simulink model "Redo7LongNoise"  (R2017b)
settings: Solver=ode45  StartTime=0.0  StopTime=MaxTime  MaxStep=timeStep  RelTol=rel  AbsTol=abs  EnableMultiTasking=on
values from neighbouring files (symbols this model uses):
  a0L = asin(min(1,(y0-yG)/l0))    [BigSweep2.m]    (also in NoiseAmbient.m; TheGoodBand.m)
  a0R = a0L-phi0    [BigSweep2.m]    (also in NoiseAmbient.m; TheGoodBand.m)
  g = 9.81    [BigSweep2.m]    (also in ElasticPendulum2.m; NoiseAmbient.m; Original_running_params.m; TheGoodBand.m)
  kL = 12000    [BigSweep2.m]    (also in NoiseAmbient.m; TheGoodBand.m)
  l0 = 1    [BigSweep2.m]    (also in ElasticPendulum2.m; NoiseAmbient.m; Original_running_params.m; TheGoodBand.m)
  m = 80    [BigSweep2.m]    (also in ElasticPendulum2.m; NoiseAmbient.m; Original_running_params.m; TheGoodBand.m)
  NoiseLevel = minNoise+(maxNoise-minNoise)*nNoise/nNoiseRuns+.00000001    [NoiseAmbient.m]    (also in TheGoodBand.m = 1e-08)
  time = now    [NoiseAmbient.m]    (also in TheGoodBand.m)
  Vx0 = real((2/m*(Esys-m*g*(y0-yG)))^.5)    [BigSweep2.m]    (also in ElasticPendulum2.m = 2.11026064741; NoiseAmbient.m = 2.11; TheGoodBand.m = 2.11)
  Vy0 = 0    [BigSweep2.m]    (also in ElasticPendulum2.m; NoiseAmbient.m; TheGoodBand.m)
  x0 = []    [AnimSMR.m]    (also in BigSweep2.m = 3; ElasticPendulum2.m = -0.2; NoiseAmbient.m = 3; Original_running_params.m = 0)
  xL0 = x0+l0*cos(a0L)    [BigSweep2.m]    (also in NoiseAmbient.m; TheGoodBand.m)
  xR0 = x0+l0*cos(a0R)    [BigSweep2.m]    (also in NoiseAmbient.m; TheGoodBand.m)
  y0 = Y0minEver+(yMaxRel-Y0minEver)*NyCycle/Ny    [BigSweep2.m]    (also in ElasticPendulum2.m = 0.98; NoiseAmbient.m = 0.98; Original_running_params.m = 1; TheGoodBand.m = 0.98)
  yG = 0    [BigSweep2.m]    (also in ElasticPendulum2.m; NoiseAmbient.m; Original_running_params.m; TheGoodBand.m)
  yL0 = y0-l0*sin(a0L)    [BigSweep2.m]    (also in NoiseAmbient.m; TheGoodBand.m)
  yR0 = y0-l0*sin(a0R)    [BigSweep2.m]    (also in NoiseAmbient.m; TheGoodBand.m)
libraries: dspswit3 x2, simulink_extras x2
settings Model: Creator=hgeyer  LastModifiedBy=jfr
settings DataIOCC: LimitDataPoints=on  SaveFormat=Array
settings OptimizationCC: ExpressionDepthLimit=2147483647  LifeSpan=inf
settings DebuggingCC: AlgebraicLoopMsg=none  UnderspecifiedInitializationDetection=Classic  MergeDetectMultiDrivingBlocksExec=none  MaxConsecutiveZCsMsg=none  SolverPrmCheckMsg=warning  StateNameClashWarn=warning  SFUnexpectedBacktrackingDiag=warning  SFNoUnconditionalDefaultTransitionDiag=warning  SFExecutionAtInitializationDiag=none
settings HardwareCC: ProdBitPerPointer=32  ProdBitPerSizeT=32  ProdBitPerPtrDiffT=32  ProdLargestAtomicFloat=None  ProdIntDivRoundTo=Undefined  ProdEndianess=Unspecified  ProdWordSize=32  ProdHWDeviceType=32-bit Generic
settings ModelReferenceCC: ModelReferenceMinAlgLoopOccurrences=on  PropagateSignalLabelsOutOfModel=off
settings CodeAppCC: StateflowObjectComments=on
settings GRTTargetCC: TargetLangStandard=C89/C90 (ANSI)  GeneratePreprocessorConditionals=Disable all
settings ConfigComp: CovMetricSettings=dw  CovHtmlReporting=on  CovSaveCumulativeToWorkspaceVar=on  CovSaveSingleToWorkspaceVar=on  CovExternalEMLEnable=off

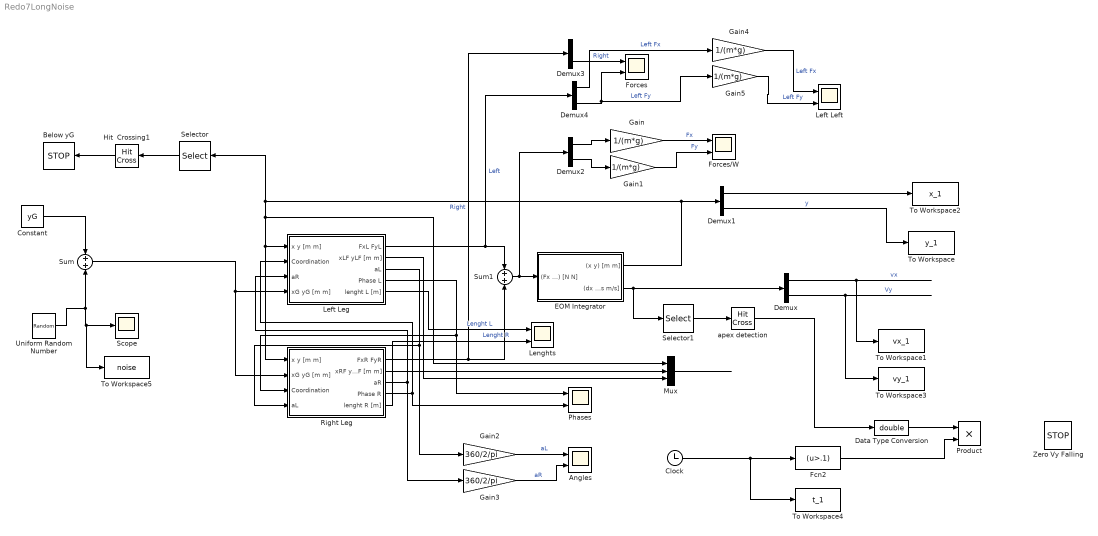
== system Redo7LongNoise ==
  "Angles " : Scope  NumInputPorts=2
  Below yG : Stop
  Clock : Clock
  Constant : Constant  Value=yG
  Data Type Conversion : DataTypeConversion  OutDataTypeStr=double
  Demux{,1..4} (5 alike) : Demux  Outputs=2
  EOM Integrator : Subsystem
  Fcn2 : Fcn  Expr=(u>.1)
  Forces : Scope  NumInputPorts=2
  Forces/W : Scope  NumInputPorts=2
  Gain{,1,4..5} (4 alike) : Gain  Gain=1/(m*g)
  Gain2 : Gain  Gain=360/2/pi
  Gain3 : Gain  Gain=360/2/pi
  Hit  Crossing1 : HitCross  HitCrossingOffset=yG  HitCrossingDirection=falling
  Left Left : Scope  NumInputPorts=2
  Left Leg : Subsystem
  Lenghts : Scope  NumInputPorts=2
  Mux : Mux  Inputs=3
  Phases : Scope  NumInputPorts=2
  Product : Product
  Right Leg : Subsystem
  Scope : Scope
  Selector : Selector  InputPortWidth=2  IndexOptions=Index vector (dialog)  Indices=2  OutputSizes=1
  Selector1 : Selector  InputPortWidth=2  IndexOptions=Index vector (dialog)  Indices=2  OutputSizes=1
  Sum : Sum
  Sum1 : Sum
  To Workspace : ToWorkspace  VariableName=y_1  SampleTime=-1
      settings: MaxDataPoints=1
  To Workspace1 : ToWorkspace  VariableName=vx_1  SampleTime=-1
      settings: MaxDataPoints=1
  To Workspace2 : ToWorkspace  VariableName=x_1  SampleTime=-1
      settings: MaxDataPoints=1
  To Workspace3 : ToWorkspace  VariableName=vy_1  SampleTime=-1
      settings: MaxDataPoints=1
  To Workspace4 : ToWorkspace  VariableName=t_1  SampleTime=-1
      settings: MaxDataPoints=1
  To Workspace5 : ToWorkspace  VariableName=noise  SampleTime=-1
  Uniform Random Number : UniformRandomNumber  Minimum=-NoiseLevel  Maximum=NoiseLevel  Seed=time  SampleTime=0.1
  Zero Vy Falling : Stop
  apex detection : HitCross  HitCrossingDirection=falling
  wires:
  Mux/1 -> ?
  Demux/2 -> To Workspace3/1  "Vy"
  Demux1/2 -> To Workspace/1  "y"
  Demux/1 -> To Workspace1/1  "vx"
  Demux1/1 -> To Workspace2/1
  Constant/1 -> Sum/1
  Left Leg/2(xLF yLF [m m]) -> Mux/3
  Sum/1 -> Left Leg/4(xG yG [m m]), Right Leg/2(xG yG [m m])
  Right Leg/2(xRF yRF [m m]) -> Mux/2
  Sum1/1 -> Demux2/1, EOM Integrator/1((Fx Fy) [N N])
  Gain/1 -> Forces/W/1  "Fx"
  Gain1/1 -> Forces/W/2  "Fy"
  Demux2/1 -> Gain/1
  Demux2/2 -> Gain1/1
  Left Leg/1(FxL FyL) -> Sum1/1, Demux4/1  "Left"
  Demux3/2 -> Forces/1  "Right"
  Gain5/1 -> Left Left/2  "Left Fy"
  Right Leg/1(FxR FyR) -> Sum1/2, Demux3/1  "Right"
  Hit  Crossing1/1 -> Below yG/1
  Selector/1 -> Hit  Crossing1/1
  EOM Integrator/1((x y) [m m]) -> Demux1/1, Right Leg/1(x y [m m]), Left Leg/1(x y [m m]), Mux/1, Selector/1
  Clock/1 -> To Workspace4/1, Fcn2/1
  apex detection/1 -> Data Type Conversion/1
  Fcn2/1 -> Product/2
  Data Type Conversion/1 -> Product/1
  Selector1/1 -> apex detection/1
  EOM Integrator/2((dx dy) [m/s m/s]) -> Selector1/1, Demux/1
  Right Leg/3(aR) -> Left Leg/3(aR), Gain3/1
  Left Leg/3(aL) -> Gain2/1, Right Leg/4(aL)
  Gain2/1 -> "Angles "/1  "aL"
  Gain3/1 -> "Angles "/2  "aR"
  Right Leg/4(Phase R) -> Phases/2, Left Leg/2(Coordination)
  Left Leg/4(Phase L) -> Right Leg/3(Coordination), Phases/1
  Left Leg/5(lenght L [m]) -> Lenghts/1  "Lenght L"
  Right Leg/5(lenght R [m]) -> Lenghts/2  "Lenght R"
  Gain4/1 -> Left Left/1  "Left Fx"
  Demux4/2 -> Gain5/1, Forces/2  "Left Fy"
  Demux4/1 -> Gain4/1  "Left Fx"
  Uniform Random Number/1 -> To Workspace5/1, Scope/1, Sum/2

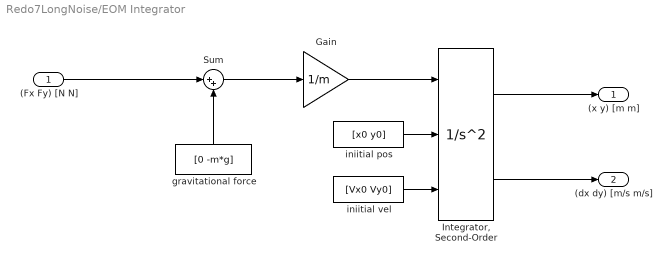
== system Redo7LongNoise/EOM Integrator ==
  (Fx Fy) [N N] : Inport
  Gain : Gain  Gain=1/m
  "Integrator, Second-Order" : SecondOrderIntegrator  ICSourceX=external  ICSourceDXDT=external
  Sum : Sum  Inputs=|++
  gravitational force : Constant  Value=[0 -m*g]
  iniitial pos : Constant  Value=[x0 y0]
  iniitial vel : Constant  Value=[Vx0 Vy0]
  (x y) [m m] : Outport
  (dx dy) [m/s m/s] : Outport  Port=2
  wires:
  Gain/1 -> "Integrator, Second-Order"/1
  iniitial vel/1 -> "Integrator, Second-Order"/3
  gravitational force/1 -> Sum/2
  (Fx Fy) [N N]/1 -> Sum/1
  iniitial pos/1 -> "Integrator, Second-Order"/2
  Sum/1 -> Gain/1
  "Integrator, Second-Order"/2 -> (dx dy) [m/s m/s]/1
  "Integrator, Second-Order"/1 -> (x y) [m m]/1

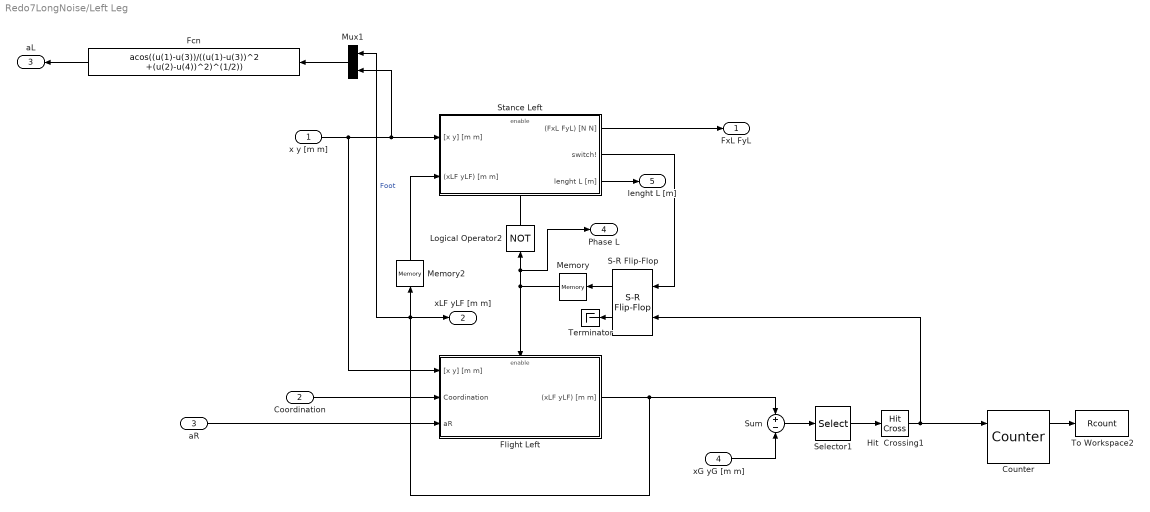
== system Redo7LongNoise/Left Leg ==
  x y [m m] : Inport
  Coordination : Inport  Port=2
  aR : Inport  Port=3
  xG yG [m m] : Inport  Port=4
  Counter : dspswit3/Counter  Direction=Up  CountEvent=Rising edge  CounterSize=User defined  MaxCount=255  InitialCount=0  Output=Count and Hit  HitValue=32  ResetInput=on  SamplesPerFrame=1  Ts=1  CntDtype=double  HitDtype=Logical
  Fcn : Fcn  Expr=acos((u(1)-u(3))/((u(1)-u(3))^2 +(u(2)-u(4))^2)^(1/2))
  Flight Left : Subsystem
  Hit  Crossing1 : HitCross  HitCrossingOffset=yG  HitCrossingDirection=falling
  Logical Operator2 : Logic  Operator=NOT  AllPortsSameDT=off  OutDataTypeStr=boolean
  Memory : Memory  InitialCondition=1
  Memory2 : Memory  InitialCondition=[xL0 yL0]
  Mux1 : Mux  Inputs=2
  S-R Flip-Flop : simulink_extras/Flip Flops/S-R Flip-Flop  initial_condition=SRleft0
  Selector1 : Selector  InputPortWidth=2  IndexOptions=Index vector (dialog)  Indices=2  OutputSizes=1
  Stance Left : Subsystem
  Sum : Sum  Inputs=+-
  Terminator : Terminator
  To Workspace2 : ToWorkspace  VariableName=Rcount  SampleTime=-1
      settings: MaxDataPoints=1
  FxL FyL : Outport
  xLF yLF [m m] : Outport  Port=2
  aL : Outport  Port=3
  Phase L : Outport  Port=4
  lenght L [m] : Outport  Port=5  InitialOutput=[0 0]
  wires:
  Mux1/1 -> Fcn/1
  Memory2/1 -> Stance Left/2((xLF yLF) [m m])
  S-R Flip-Flop/1 -> Memory/1
  Stance Left/1((FxL FyL) [N N]) -> FxL FyL/1
  Stance Left/2(switch!) -> S-R Flip-Flop/1
  Logical Operator2/1 -> Stance Left/Enable
  S-R Flip-Flop/2 -> Terminator/1
  x y [m m]/1 -> Mux1/2, Stance Left/1("[x y] [m m]"), Flight Left/1("[x y] [m m]")
  aR/1 -> Flight Left/3(aR)
  Coordination/1 -> Flight Left/2(Coordination)
  Stance Left/3(lenght L [m]) -> lenght L [m]/1
  Memory/1 -> Flight Left/Enable, Phase L/1, Logical Operator2/1
  Fcn/1 -> aL/1
  Sum/1 -> Selector1/1
  Flight Left/1(" (xLF yLF) [m m]") -> Sum/1, xLF yLF [m m]/1, Memory2/1, Mux1/1  "Foot"
  xG yG [m m]/1 -> Sum/2
  Selector1/1 -> Hit  Crossing1/1
  Counter/1 -> To Workspace2/1
  Hit  Crossing1/1 -> Counter/1, S-R Flip-Flop/2

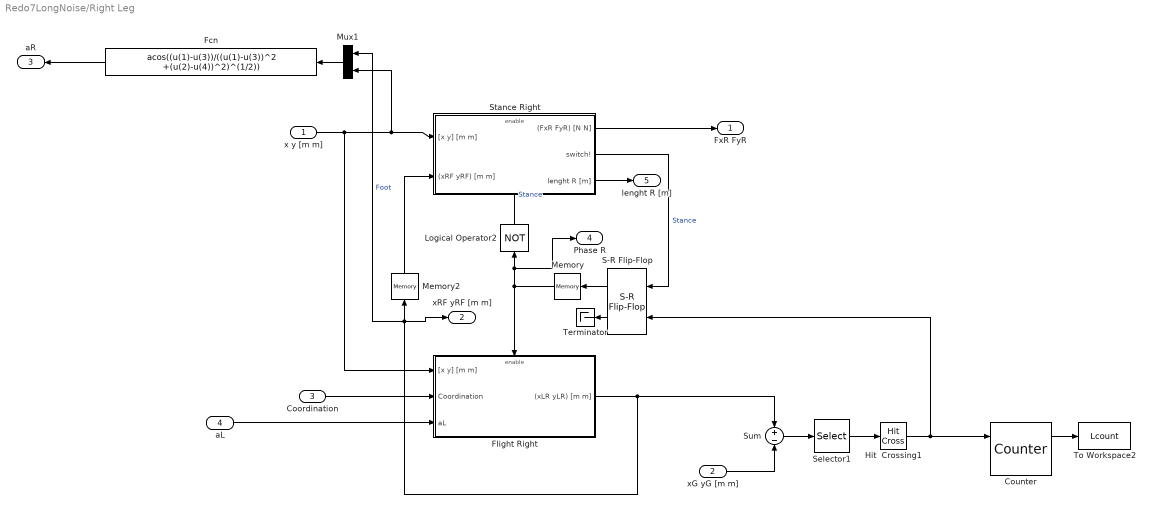
== system Redo7LongNoise/Right Leg ==
  x y [m m] : Inport
  xG yG [m m] : Inport  Port=2
  Coordination : Inport  Port=3
  aL : Inport  Port=4
  Counter : dspswit3/Counter  Direction=Up  CountEvent=Rising edge  CounterSize=User defined  MaxCount=255  InitialCount=0  Output=Count and Hit  HitValue=32  ResetInput=on  SamplesPerFrame=1  Ts=1  CntDtype=double  HitDtype=Logical
  Fcn : Fcn  Expr=acos((u(1)-u(3))/((u(1)-u(3))^2 +(u(2)-u(4))^2)^(1/2))
  Flight Right : Subsystem
  Hit  Crossing1 : HitCross  HitCrossingOffset=yG  HitCrossingDirection=falling
  Logical Operator2 : Logic  Operator=NOT  AllPortsSameDT=off  OutDataTypeStr=boolean
  Memory : Memory  InitialCondition=1
  Memory2 : Memory  InitialCondition=[xR0 yR0]
  Mux1 : Mux  Inputs=2
  S-R Flip-Flop : simulink_extras/Flip Flops/S-R Flip-Flop  initial_condition=SRright0
  Selector1 : Selector  InputPortWidth=2  IndexOptions=Index vector (dialog)  Indices=2  OutputSizes=1
  Stance Right : Subsystem
  Sum : Sum  Inputs=+-
  Terminator : Terminator
  To Workspace2 : ToWorkspace  VariableName=Lcount  SampleTime=-1
      settings: MaxDataPoints=1
  FxR FyR : Outport
  xRF yRF [m m] : Outport  Port=2
  aR : Outport  Port=3
  Phase R : Outport  Port=4
  lenght R [m] : Outport  Port=5  InitialOutput=[0 0]
  wires:
  Mux1/1 -> Fcn/1
  Memory2/1 -> Stance Right/2((xRF yRF) [m m])
  S-R Flip-Flop/1 -> Memory/1
  Stance Right/1((FxR FyR) [N N]) -> FxR FyR/1
  Stance Right/2(switch!) -> S-R Flip-Flop/1  "Stance"
  S-R Flip-Flop/2 -> Terminator/1
  x y [m m]/1 -> Flight Right/1("[x y] [m m]"), Mux1/2, Stance Right/1("[x y] [m m]")
  aL/1 -> Flight Right/3(aL)
  Coordination/1 -> Flight Right/2(Coordination)
  Fcn/1 -> aR/1
  Stance Right/3(lenght R [m]) -> lenght R [m]/1
  Logical Operator2/1 -> Stance Right/Enable  "Stance"
  Memory/1 -> Flight Right/Enable, Phase R/1, Logical Operator2/1
  Sum/1 -> Selector1/1
  Flight Right/1(" (xLR yLR) [m m]") -> Sum/1, xRF yRF [m m]/1, Memory2/1, Mux1/1  "Foot"
  Selector1/1 -> Hit  Crossing1/1
  Hit  Crossing1/1 -> Counter/1, S-R Flip-Flop/2
  xG yG [m m]/1 -> Sum/2
  Counter/1 -> To Workspace2/1

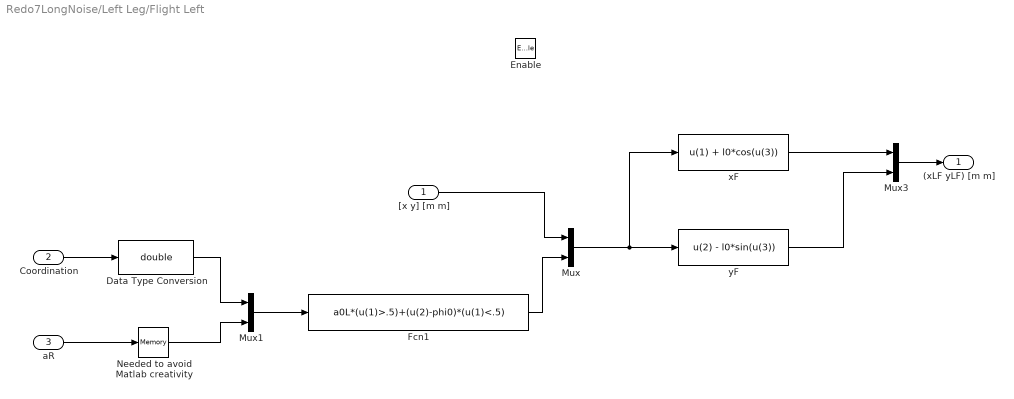
== system Redo7LongNoise/Left Leg/Flight Left ==
  "[x y] [m m]" : Inport
  Coordination : Inport  Port=2
  aR : Inport  Port=3
  Enable : EnablePort  StatesWhenEnabling=reset
  Data Type Conversion : DataTypeConversion  OutDataTypeStr=double
  Fcn1 : Fcn  Expr=a0L*(u(1)>.5)+(u(2)-phi0)*(u(1)<.5)
  Mux : Mux  Inputs=2
  Mux1 : Mux  Inputs=2
  Mux3 : Mux  Inputs=2
  Needed to avoid Matlab creativity : Memory  InitialCondition=a0L
  xF : Fcn  Expr=u(1) + l0*cos(u(3))
  yF : Fcn  Expr=u(2) - l0*sin(u(3))
  " (xLF yLF) [m m]" : Outport  InitialOutput=[0 0]
  wires:
  Mux3/1 -> " (xLF yLF) [m m]"/1
  xF/1 -> Mux3/1
  "[x y] [m m]"/1 -> Mux/1
  Mux/1 -> xF/1, yF/1
  Fcn1/1 -> Mux/2
  Data Type Conversion/1 -> Mux1/1
  Coordination/1 -> Data Type Conversion/1
  yF/1 -> Mux3/2
  Mux1/1 -> Fcn1/1
  aR/1 -> Needed to avoid Matlab creativity/1
  Needed to avoid Matlab creativity/1 -> Mux1/2

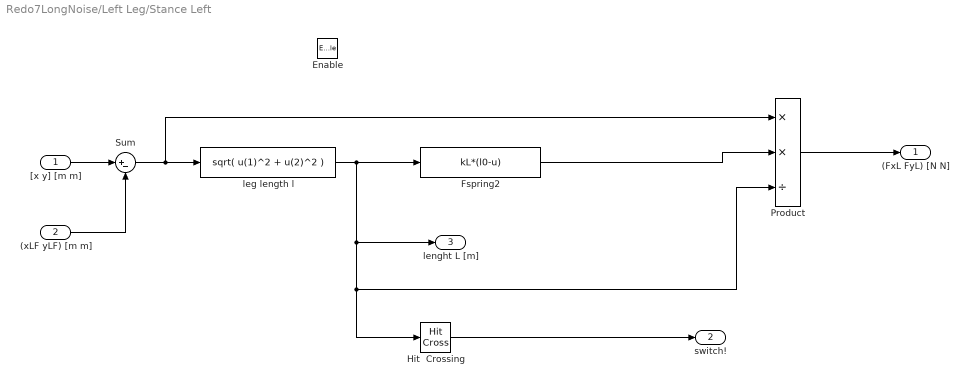
== system Redo7LongNoise/Left Leg/Stance Left ==
  "[x y] [m m]" : Inport
  (xLF yLF) [m m] : Inport  Port=2
  Enable : EnablePort  StatesWhenEnabling=reset
  Fspring2 : Fcn  Expr=kL*(l0-u)
  Hit  Crossing : HitCross  HitCrossingOffset=l0  HitCrossingDirection=rising
  Product : Product  Inputs=**/  RndMeth=Zero
  Sum : Sum  Inputs=|+-
  leg length l : Fcn  Expr=sqrt( u(1)^2 + u(2)^2 )
  (FxL FyL) [N N] : Outport  OutputWhenDisabled=reset  InitialOutput=[0 0]
  switch! : Outport  Port=2  OutputWhenDisabled=reset  InitialOutput=0
  lenght L [m] : Outport  Port=3  InitialOutput=((x0-xL0)^2+(y0-yL0)^2)^(1/2)
  wires:
  Sum/1 -> Product/1, leg length l/1
  "[x y] [m m]"/1 -> Sum/1
  Product/1 -> (FxL FyL) [N N]/1
  Hit  Crossing/1 -> switch!/1
  Fspring2/1 -> Product/2
  leg length l/1 -> Fspring2/1, lenght L [m]/1, Hit  Crossing/1, Product/3
  (xLF yLF) [m m]/1 -> Sum/2

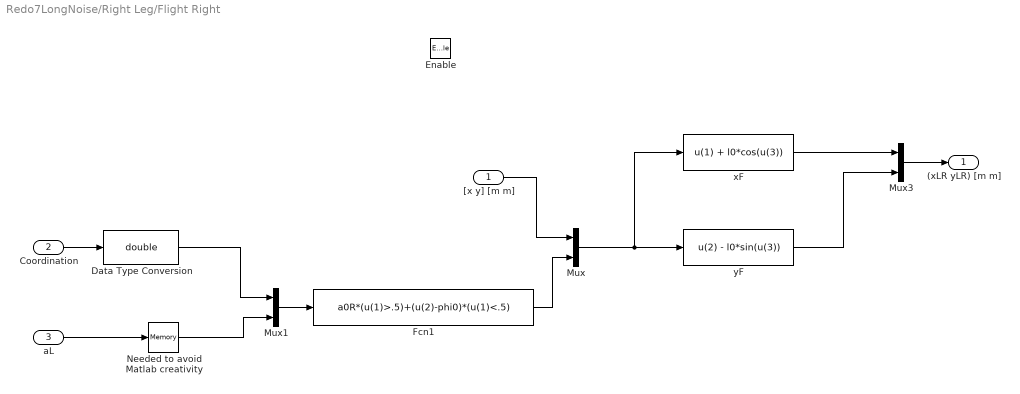
== system Redo7LongNoise/Right Leg/Flight Right ==
  "[x y] [m m]" : Inport
  Coordination : Inport  Port=2
  aL : Inport  Port=3
  Enable : EnablePort  StatesWhenEnabling=reset
  Data Type Conversion : DataTypeConversion  OutDataTypeStr=double
  Fcn1 : Fcn  Expr=a0R*(u(1)>.5)+(u(2)-phi0)*(u(1)<.5)
  Mux : Mux  Inputs=2
  Mux1 : Mux  Inputs=2
  Mux3 : Mux  Inputs=2
  "Needed to avoid Matlab creativity " : Memory  InitialCondition=a0R
  xF : Fcn  Expr=u(1) + l0*cos(u(3))
  yF : Fcn  Expr=u(2) - l0*sin(u(3))
  " (xLR yLR) [m m]" : Outport  InitialOutput=[0 0]
  wires:
  Mux3/1 -> " (xLR yLR) [m m]"/1
  xF/1 -> Mux3/1
  "[x y] [m m]"/1 -> Mux/1
  Mux/1 -> xF/1, yF/1
  Fcn1/1 -> Mux/2
  Coordination/1 -> Data Type Conversion/1
  yF/1 -> Mux3/2
  Mux1/1 -> Fcn1/1
  aL/1 -> "Needed to avoid Matlab creativity "/1
  Data Type Conversion/1 -> Mux1/1
  "Needed to avoid Matlab creativity "/1 -> Mux1/2

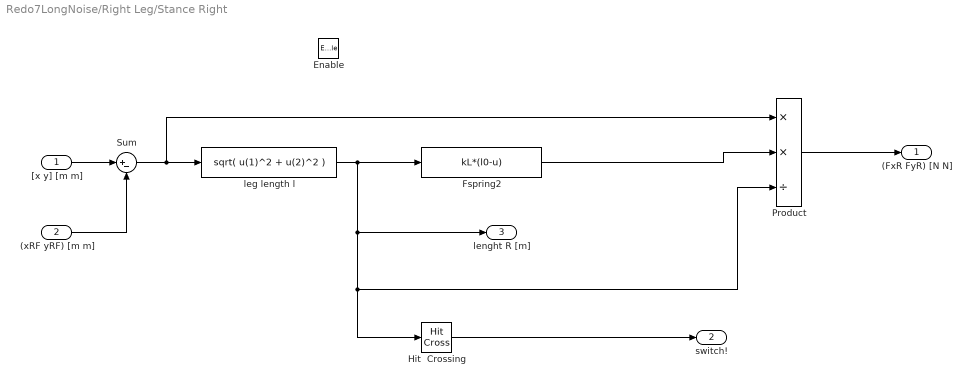
== system Redo7LongNoise/Right Leg/Stance Right ==
  "[x y] [m m]" : Inport
  (xRF yRF) [m m] : Inport  Port=2
  Enable : EnablePort  StatesWhenEnabling=reset
  Fspring2 : Fcn  Expr=kL*(l0-u)
  Hit  Crossing : HitCross  HitCrossingOffset=l0  HitCrossingDirection=rising
  Product : Product  Inputs=**/  RndMeth=Zero
  Sum : Sum  Inputs=|+-
  leg length l : Fcn  Expr=sqrt( u(1)^2 + u(2)^2 )
  (FxR FyR) [N N] : Outport  OutputWhenDisabled=reset  InitialOutput=[0 0]
  switch! : Outport  Port=2  OutputWhenDisabled=reset  InitialOutput=0
  lenght R [m] : Outport  Port=3  InitialOutput=((x0-xR0)^2+(y0-yR0)^2)^(1/2)
  wires:
  Sum/1 -> Product/1, leg length l/1
  "[x y] [m m]"/1 -> Sum/1
  Product/1 -> (FxR FyR) [N N]/1
  Hit  Crossing/1 -> switch!/1
  Fspring2/1 -> Product/2
  leg length l/1 -> Fspring2/1, lenght R [m]/1, Hit  Crossing/1, Product/3
  (xRF yRF) [m m]/1 -> Sum/2
